simulink model "SatelliteServicing_Mission"  (R2023a)
settings: Solver=FixedStepAuto  StartTime=0.0  StopTime=endTime  FixedStep=stepSize  RelTol=1e-3  EnableMultiTasking=on
values from neighbouring files (symbols this model uses):
  nsat = 4    [loadCubesatParams.m]
undefined symbols (not defined in the file or in its folder): arm, client, cubesat, orbit, smiData, X, Y, Z
libraries: nesl_utility x53, sm_lib x32
(part 1 of 2)
settings Model: Creator=Andy  LastModifiedBy=Andy
settings SolverCC: PositivePriorityOrder=on
settings OptimizationCC: EnhancedBackFolding=on  PassReuseOutputArgsAs=Individual arguments  OptimizeBlockOrder=speed  DifferentSizesBufferReuse=on  OptimizationCustomize=off  EfficientTunableParamExpr=on
settings DebuggingCC: ParameterTunabilityLossMsg=error  UnconnectedInputMsg=warning  UnconnectedOutputMsg=warning  UnconnectedLineMsg=warning
settings ModelReferenceCC: EnableRefExpFcnMdlSchedulingChecks=on
settings SFSimCC: MATLABDynamicMemAlloc=off  SimTargetLang=C++
settings RTWCC: Description=Embedded Coder  SystemTargetFile=ert.tlc  GenCodeOnly=on  PackageGeneratedCodeAndArtifacts=on  TemplateMakefile=ert_default_tmf  GenerateReport=on  Toolchain=GNU GCC Embedded Linux  BuildConfiguration=Faster Runs  LaunchReport=on  TargetLang=C++  DLArmComputeVersion=19.05
settings CodeAppCC: ForceParamTrailComments=on  IgnoreCustomStorageClasses=off  OperatorAnnotations=on  SimulinkDataObjDesc=on  SFDataObjDesc=on  InsertBlockDesc=on
settings ERTTargetCC: TargetLangStandard=C++11 (ISO)  UtilityFuncGeneration=Shared location  GenerateSampleERTMain=on  CodeInterfacePackaging=Reusable function  SupportContinuousTime=on  SupportVariableSizeSignals=on  GenerateAllocFcn=on  RootIOFormat=Structure reference  ERTCustomFileTemplate=example_file_process.tlc
settings SimscapeCC: SimscapeLogType=all

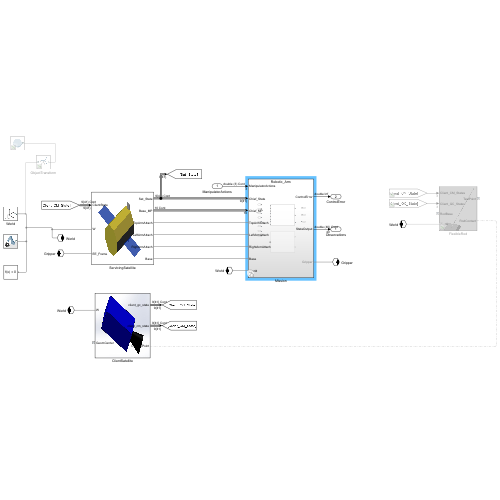
[thumbnail: Simulink's stored preview of the top-level diagram]
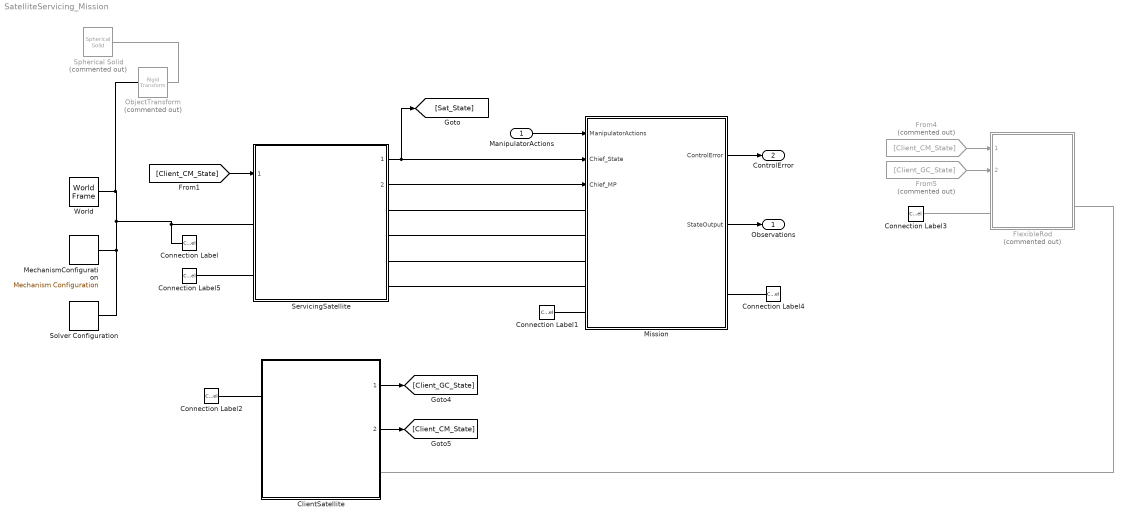
== system SatelliteServicing_Mission ==
  ManipulatorActions : Inport  PortDimensions=nAction
  ClientSatellite : Subsystem  ReferencedSubsystem=ClientSatellite
  Connection Label{,1..3} (4 alike) : ConnectionLabel  Label=World
  Connection Label4 : ConnectionLabel  Label=Gripper
  Connection Label5 : ConnectionLabel  Label=Gripper
  FlexibleRod : Subsystem  Commented=on  ReferencedSubsystem=FlexibleRodModel
  From4 : From  Commented=on  GotoTag=Client_CM_State
  From5 : From  Commented=on  GotoTag=Client_GC_State
  MechanismConfiguration : sm_lib/Utilities/Mechanism Configuration  UniformGravity=Constant  GravityVector=[0 0 -9.80665]*0  GravityVectorUnits=m/s^2  LinearizationDelta=0.001  JointModeTransitionNonlinearIterations=2
  Mission : Subsystem  Variant=on  VariantControl=Choice
  ObjectTransform : sm_lib/Frames and Transforms/Rigid Transform  Commented=on  TranslationMethod=Cartesian  TranslationStandardOffset=0  TranslationStandardOffsetUnits=m  TranslationStandardAxis=+Z  TranslationCartesianOffset=[0 -0.6 0]  TranslationCartesianOffsetUnits=m  TranslationROffset=0  TranslationROffsetUnits=m  TranslationZOffset=0  TranslationZOffsetUnits=m  TranslationThetaOffset=0  TranslationThetaOffsetUnits=deg  RotationMethod=None  RotationAngleUnits=rad  RotationStandardAxis=+Z  RotationAngle=smiData.RigidTransform(21).angle  RotationArbitraryAxis=smiData.RigidTransform(21).axis  FollAlignAxisA=+X  BaseAlignAxisA=+Y  FollAlignAxisB=+Y  BaseAlignAxisB=+Z  RotationSequenceAxes=FollowerAxes  RotationSequence=XYZ  RotationSequenceAngles=[0 0 0]  RotationSequenceAnglesUnits=rad  RotationMatrix=[1 0 0; 0 1 0; 0 0 1]  Quaternion=[1 0 0 0]
  ServicingSatellite : Subsystem  ReferencedSubsystem=ServicingSatellite
  Solver Configuration : nesl_utility/Solver Configuration  PhysicalDomain=network_engine_domain  SubClassName=solver  LeftPortType=input  RightPortType=generic  Tones=[]  Harmonics=[]  SimulateNoise=off  Profile=off  UseLocalSampling=off  EnableSwitchedLinearOptims=on  FrequencyDomain=off  UseCCode=off  RelTol=0.001  AbsTol=1e-06  MinStep=1e-09  ToWorkspace=off  RevertToSquareIcSolve=off  NumHomotopyIterations=100  PhasorMode=off  PhasorModeNumHarmonics=1  ConsistencySolver=NEWTON_FTOL  IndexReductionMethod=DerivativeReplacement  DoDC=off  ResidualTolerance=1e-09  ConsistencyTolSource=GLOBAL  ConsistencyAbsTol=0.001  ConsistencyRelTol=0.001  ConsistencyTolFactor=0.001  UseLocalSolver=off  LocalSolverChoice=NE_BACKWARD_EULER_ADVANCER  ResolveIndetEquations=on  FunctionEvalNumThread=1  LocalSolverSampleTime=0.001  DoFixedCost=off  MaxNonlinIter=3  MaxModeIter=2  ComputeImpulses=off  ImpulseIterations=2  LinearAlgebra=auto  LinearAlgebraNumThread=0  EquationFormulation=NE_TIME_EF  DelaysMemoryBudget=1024  AutomaticFiltering=on  FilteringTimeConstant=0.001  PartitionStorageMethod=AS_NEEDED  PartitionMemoryBudget=1024  PartitionMethod=ROBUST
  Spherical Solid : sm_lib/Body Elements/Spherical Solid  Commented=on  GraphicAmbientColor=[0.15 0.15 0.15 1.0]  BasedOnType=Density  CenterOfMass=[0 0 0]  CenterOfMassUnits=m  GraphicDiffuseColor=[0.5 0.5 0.5]  Density=1000  DensityUnits=kg/m^3  DoExposeReferenceFrame=on  GraphicEmissiveColor=[0.0 0.0 0.0 1.0]  ExportEntireGeometry=off  SerializedExposedGeometries=<ExposedGeometries/>  SerializedFrames=<Frames/>  MarkerShape=Sphere  MarkerSize=10  GraphicType=FromGeometry  InertiaType=CalculateFromGeometry  Mass=1  MassUnits=kg  MomentsOfInertia=[1 1 1]  MomentsOfInertiaUnits=kg*m^2  GraphicOpacity=1.0  ProductsOfInertia=[0 0 0]  ProductsOfInertiaUnits=kg*m^2  GraphicShininess=75  GraphicSpecularColor=[0.5 0.5 0.5 1.0]  SphereRadius=0.1  SphereRadiusUnits=m  GraphicVisPropType=SimpleVisualProperties
  World : sm_lib/Frames and Transforms/World Frame
  Observations : Outport
  ControlError : Outport  Port=2
  wires:
  ServicingSatellite/1 -> [Sat_State], Mission/2(Chief_State)
  ClientSatellite/1 -> [Client_GC_State]
  ClientSatellite/2 -> [Client_CM_State]
  ManipulatorActions/1 -> Mission/1(ManipulatorActions)
  Mission/1(ControlError) -> ControlError/1
  Mission/2(StateOutput) -> Observations/1
  From5/1 -> FlexibleRod/2
  From4/1 -> FlexibleRod/1
  [Client_CM_State] -> ServicingSatellite/1
  ServicingSatellite/2 -> Mission/3(Chief_MP)
  connections:
  MechanismConfiguration/RConn1 -- ServicingSatellite/LConn1 -- Connection Label/LConn1 -- ObjectTransform/LConn1 -- World/RConn1 -- Solver Configuration/RConn1
  FlexibleRod/RConn2 -- ClientSatellite/RConn1
  Connection Label2/LConn1 -- ClientSatellite/LConn1
  FlexibleRod/LConn2 -- Connection Label3/LConn1
  Mission/LConn1 -- ServicingSatellite/RConn1
  Mission/LConn4 -- ServicingSatellite/RConn4
  Mission/LConn5 -- Connection Label1/LConn1
  Connection Label4/LConn1 -- Mission/RConn1
  Connection Label5/LConn1 -- ServicingSatellite/LConn2
  ServicingSatellite/RConn2 -- Mission/LConn2
  ServicingSatellite/RConn3 -- Mission/LConn3
  Spherical Solid/RConn1 -- ObjectTransform/RConn1

== system SatelliteServicing_Mission/Mission ==
  ManipulatorActions : Inport
  Chief_State : Inport  Port=2
  Chief_MP : Inport  Port=3
  Cubesat_Inspection : Subsystem  VariantControl=VSS_CubeSatOperation
  Robotic_Arm : Subsystem  VariantControl=VSS_RoboticArmOperation
  Gripper : PMIOPort  Side=Right
  TopArmAttach : PMIOPort  Port=2  Side=Left
  LeftArmAttach : PMIOPort  Port=3  Side=Left
  RightArmAttach : PMIOPort  Port=4  Side=Left
  Base : PMIOPort  Port=5  Side=Left
  World : PMIOPort  Port=6  Side=Left
  ControlError : Outport
  StateOutput : Outport  Port=2

== system SatelliteServicing_Mission/Mission/Cubesat_Inspection ==
  Bus Selector : BusSelector  OutputSignals=Cubesat1_RelState.Rel_Position,Cubesat1_RelState.Rel_Velocity,Cubesat1_RelState.Rel_Acceleration,Cubesat2_RelState.Rel_Position,Cubesat2_RelState.Rel_Velocity,Cubesat2_RelState.Rel_Acceleration,Cubesat3_RelState.Rel_Position,Cubesat3_RelState.Rel_Velocity,Cubesat3_RelState.Rel_Acceleration,Cubesat4_RelState.Rel_Position,Cubesat4_RelState.Rel_Velocity,Cubesat4_RelState.Rel_Acceleration
  Cubesats : Subsystem
  InspectionCoverage : Subsystem
  Mux1 : Mux  Inputs=12
  To Workspace1 : ToWorkspace  VariableName=cubesatRelState  SaveFormat=Timeseries  SampleTime=-1
  World : PMIOPort  Side=Left
  StateOutput : Outport
  ControlError : Outport  Port=2
  wires:
  Cubesats/1(Cubesat_RelState) -> Bus Selector/1, To Workspace1/1, InspectionCoverage/1(relative_state)
  InspectionCoverage/1(coverageCredit) -> ControlError/1
  Mux1/1 -> StateOutput/1
  Bus Selector/1 -> Mux1/1  "<Rel_Position>"
  Bus Selector/2 -> Mux1/2  "<Rel_Velocity>"
  Bus Selector/3 -> Mux1/3  "<Rel_Acceleration>"
  Bus Selector/4 -> Mux1/4  "<Rel_Position>"
  Bus Selector/5 -> Mux1/5  "<Rel_Velocity>"
  Bus Selector/6 -> Mux1/6  "<Rel_Acceleration>"
  Bus Selector/7 -> Mux1/7  "<Rel_Position>"
  Bus Selector/8 -> Mux1/8  "<Rel_Velocity>"
  Bus Selector/9 -> Mux1/9  "<Rel_Acceleration>"
  Bus Selector/10 -> Mux1/10  "<Rel_Position>"
  Bus Selector/11 -> Mux1/11  "<Rel_Velocity>"
  Bus Selector/12 -> Mux1/12  "<Rel_Acceleration>"
  connections:
  World/RConn1 -- Cubesats/LConn1

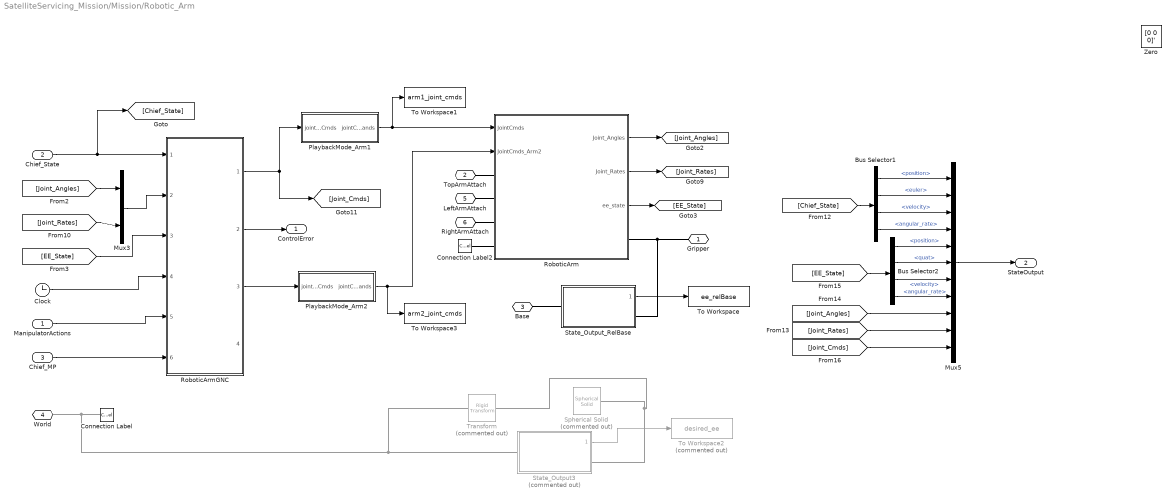
== system SatelliteServicing_Mission/Mission/Robotic_Arm ==
  ManipulatorActions : Inport  PortDimensions=nAction
  Chief_State : Inport  Port=2
  Chief_MP : Inport  Port=3
  Bus Selector1 : BusSelector  OutputSignals=translation.position,rotation.euler,translation.velocity,rotation.angular_rate
  Bus Selector2 : BusSelector  OutputSignals=translation.position,rotation.quat,translation.velocity,rotation.angular_rate
  Clock : Clock
  Connection Label : ConnectionLabel  Label=World
  Connection Label2 : ConnectionLabel  Label=World
  Mux3 : Mux  Inputs=2
  Mux5 : Mux  Inputs=11
  PlaybackMode_Arm1 : Subsystem  Variant=on  VariantControl=Choice
  PlaybackMode_Arm2 : Subsystem  Variant=on  VariantControl=Choice
  RoboticArm : Subsystem  Variant=on  VariantControl=Choice
  RoboticArmGNC : Subsystem  SystemSampleTime=0.001  ReferencedSubsystem=RoboticArmGNC
      settings: MinAlgLoopOccurrences=on
  Spherical Solid : sm_lib/Body Elements/Spherical Solid  Commented=on  GraphicAmbientColor=[0.15 0.15 0.15 1.0]  BasedOnType=Density  CenterOfMass=[0 0 0]  CenterOfMassUnits=m  GraphicDiffuseColor=[1.0 0.0 0.0]  Density=1000  DensityUnits=kg/m^3  DoExposeReferenceFrame=on  GraphicEmissiveColor=[0.0 0.0 0.0 1.0]  ExportEntireGeometry=off  SerializedExposedGeometries=<ExposedGeometries/>  SerializedFrames=<Frames/>  MarkerShape=Sphere  MarkerSize=10  GraphicType=FromGeometry  InertiaType=CalculateFromGeometry  Mass=1  MassUnits=kg  MomentsOfInertia=[1 1 1]  MomentsOfInertiaUnits=kg*m^2  GraphicOpacity=1.0  ProductsOfInertia=[0 0 0]  ProductsOfInertiaUnits=kg*m^2  GraphicShininess=75  GraphicSpecularColor=[0.5 0.5 0.5 1.0]  SphereRadius=0.01  SphereRadiusUnits=m  GraphicVisPropType=SimpleVisualProperties
  State_Output3 : Subsystem  Commented=on  ReferencedSubsystem=Collect_State_Output
  State_Output_RelBase : Subsystem  ReferencedSubsystem=Collect_State_Output_BaseFrame
  To Workspace : ToWorkspace  VariableName=ee_relBase  SaveFormat=Timeseries  SampleTime=-1
  To Workspace1 : ToWorkspace  VariableName=arm1_joint_cmds  SaveFormat=Timeseries  SampleTime=-1
  To Workspace2 : ToWorkspace  Commented=on  VariableName=desired_ee  SaveFormat=Timeseries  SampleTime=-1
  To Workspace3 : ToWorkspace  VariableName=arm2_joint_cmds  SaveFormat=Timeseries  SampleTime=-1
  Transform : sm_lib/Frames and Transforms/Rigid Transform  Commented=on  TranslationMethod=Cartesian  TranslationStandardOffset=0  TranslationStandardOffsetUnits=mm  TranslationStandardAxis=+Z  TranslationCartesianOffset=desired_ee_world_pos  TranslationCartesianOffsetUnits=m  TranslationROffset=0  TranslationROffsetUnits=m  TranslationZOffset=0  TranslationZOffsetUnits=m  TranslationThetaOffset=0  TranslationThetaOffsetUnits=deg  RotationMethod=RotationSequence  RotationAngleUnits=rad  RotationStandardAxis=+Z  RotationAngle=arm(1).smiData.RigidTransform(2).angle  RotationArbitraryAxis=desired_  FollAlignAxisA=+X  BaseAlignAxisA=+Y  FollAlignAxisB=+Y  BaseAlignAxisB=+Z  RotationSequenceAxes=FollowerAxes  RotationSequence=XYZ  RotationSequenceAngles=desired_ee_world_ori  RotationSequenceAnglesUnits=rad  RotationMatrix=[1 0 0; 0 1 0; 0 0 1]  Quaternion=[1 0 0 0]
  Zero : Constant  Value=[0 0 0]'
  Gripper : PMIOPort  Side=Right
  TopArmAttach : PMIOPort  Port=2  Side=Left
  Base : PMIOPort  Port=3  Side=Left
  World : PMIOPort  Port=4  Side=Left
  LeftArmAttach : PMIOPort  Port=5  Side=Left
  RightArmAttach : PMIOPort  Port=6  Side=Left
  ControlError : Outport
  StateOutput : Outport  Port=2
  wires:
  RoboticArm/2(Joint_Rates) -> [Joint_Rates]
  Chief_State/1 -> [Chief_State], RoboticArmGNC/1
  RoboticArm/3(ee_state) -> [EE_State]
  RoboticArm/1(Joint_Angles) -> [Joint_Angles]
  ManipulatorActions/1 -> RoboticArmGNC/5
  State_Output_RelBase/1 -> To Workspace/1
  [EE_State] -> RoboticArmGNC/3
  Clock/1 -> RoboticArmGNC/4
  RoboticArmGNC/2 -> ControlError/1
  PlaybackMode_Arm1/1(jointCommands) -> RoboticArm/1(JointCmds), To Workspace1/1
  Bus Selector1/1 -> Mux5/1  "<position>"
  [Joint_Cmds] -> Mux5/11
  [Joint_Angles] -> Mux5/9
  Bus Selector2/1 -> Mux5/5  "<position>"
  Bus Selector1/3 -> Mux5/3  "<velocity>"
  Bus Selector1/2 -> Mux5/2  "<euler>"
  Bus Selector1/4 -> Mux5/4  "<angular_rate>"
  Bus Selector2/2 -> Mux5/6  "<quat>"
  Bus Selector2/4 -> Mux5/8  "<angular_rate>"
  Mux5/1 -> StateOutput/1
  Bus Selector2/3 -> Mux5/7  "<velocity>"
  [Chief_State] -> Bus Selector1/1
  [Joint_Rates] -> Mux5/10
  [EE_State] -> Bus Selector2/1
  Chief_MP/1 -> RoboticArmGNC/6
  RoboticArmGNC/1 -> [Joint_Cmds], PlaybackMode_Arm1/1(jointTorqueCmds)
  State_Output3/1 -> To Workspace2/1
  RoboticArmGNC/3 -> PlaybackMode_Arm2/1(jointTorqueCmds)
  PlaybackMode_Arm2/1(jointCommands) -> To Workspace3/1, RoboticArm/2(JointCmds_Arm2)
  [Joint_Angles] -> Mux3/1
  [Joint_Rates] -> Mux3/2
  Mux3/1 -> RoboticArmGNC/2
  connections:
  State_Output_RelBase/RConn1 -- RoboticArm/RConn1 -- Gripper/RConn1
  Base/RConn1 -- State_Output_RelBase/LConn1
  RoboticArm/LConn1 -- TopArmAttach/RConn1
  Connection Label2/LConn1 -- RoboticArm/LConn4
  LeftArmAttach/RConn1 -- RoboticArm/LConn2
  RightArmAttach/RConn1 -- RoboticArm/LConn3
  State_Output3/LConn1 -- Connection Label/LConn1 -- World/RConn1 -- Transform/LConn1
  State_Output3/RConn1 -- Transform/RConn1 -- Spherical Solid/RConn1

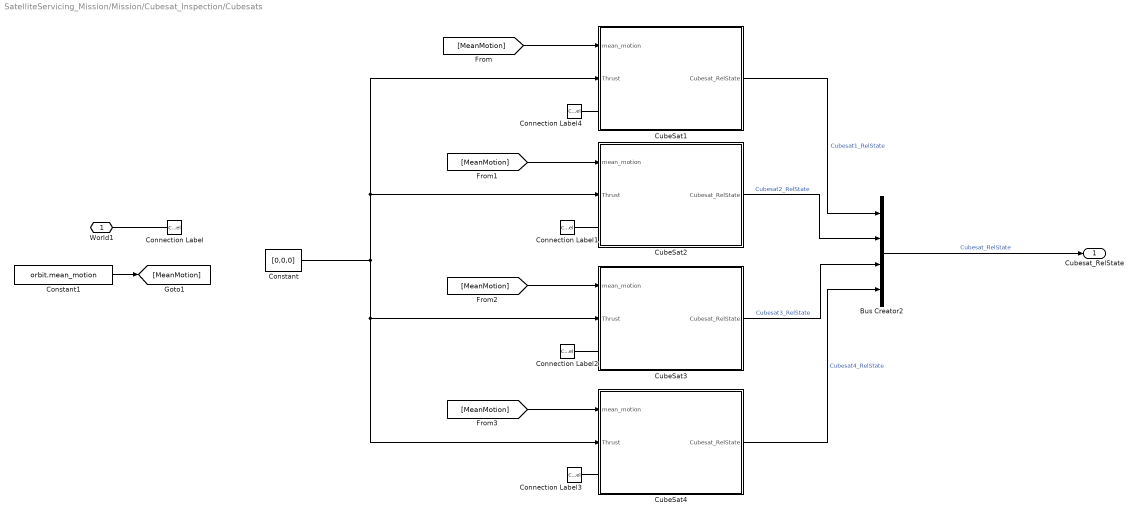
== system SatelliteServicing_Mission/Mission/Cubesat_Inspection/Cubesats ==
  Bus Creator2 : BusCreator  Inputs=4
  Connection Label{,1..4} (5 alike) : ConnectionLabel  Label=World
  Constant : Constant  Value=[0,0,0]
  Constant1 : Constant  Value=orbit.mean_motion
  CubeSat1 : Subsystem  Variant=on  VariantControl=Choice  AllowZeroVariantControls=on
  CubeSat2 : Subsystem  Variant=on  VariantControl=Choice  AllowZeroVariantControls=on
  CubeSat3 : Subsystem  Variant=on  VariantControl=Choice  AllowZeroVariantControls=on
  CubeSat4 : Subsystem  Variant=on  VariantControl=Choice  AllowZeroVariantControls=on
  World1 : PMIOPort  Side=Left
  Cubesat_RelState : Outport
  wires:
  CubeSat3/1(Cubesat_RelState) -> Bus Creator2/3  "Cubesat3_RelState"
  Constant1/1 -> [MeanMotion]
  CubeSat2/1(Cubesat_RelState) -> Bus Creator2/2  "Cubesat2_RelState"
  CubeSat4/1(Cubesat_RelState) -> Bus Creator2/4  "Cubesat4_RelState"
  [MeanMotion] -> CubeSat3/1(mean_motion)
  [MeanMotion] -> CubeSat4/1(mean_motion)
  Bus Creator2/1 -> Cubesat_RelState/1  "Cubesat_RelState"
  CubeSat1/1(Cubesat_RelState) -> Bus Creator2/1  "Cubesat1_RelState"
  Constant/1 -> CubeSat1/2(Thrust), CubeSat2/2(Thrust), CubeSat4/2(Thrust), CubeSat3/2(Thrust)
  [MeanMotion] -> CubeSat1/1(mean_motion)
  [MeanMotion] -> CubeSat2/1(mean_motion)
  connections:
  Connection Label2/LConn1 -- CubeSat3/LConn1
  World1/RConn1 -- Connection Label/LConn1
  Connection Label4/LConn1 -- CubeSat1/LConn1
  Connection Label3/LConn1 -- CubeSat4/LConn1
  Connection Label1/LConn1 -- CubeSat2/LConn1

== system SatelliteServicing_Mission/Mission/Cubesat_Inspection/InspectionCoverage ==
  relative_state : Inport
  Constant1 : Constant  Value=nsat
  Constant2 : Constant  Value=client.inspectionFOV
  Constant3 : Constant  Value=client.faceCenter
  Constant4 : Constant  Value=zeros(client.nFaces,1)  VectorParams1D=off
  Constant5 : Constant  Value=client.faceRadius
  Constant6 : Constant  Value=client.inspectionSphereRadius
  Delay : Delay  DelayLength=1  InitialConditionSource=Input port
      settings: InputPortMap=u0,p4
  Delay1 : Delay  DelayLength=1  InitialConditionSource=Input port
      settings: InputPortMap=u0,p4
  Reshape : Reshape  OutputDimensionality=Column vector (2-D)
  To Workspace7 : ToWorkspace  VariableName=coverageOut  SaveFormat=Timeseries  SampleTime=-1
  To Workspace8 : ToWorkspace  VariableName=creditOut  SaveFormat=Timeseries  SampleTime=-1
  computeCoverage : MATLAB Function  TreatAsAtomicUnit=on
  coverageCredit : Outport
  wires:
  computeCoverage/2(credit_out) -> To Workspace8/1, Delay1/1, coverageCredit/1
  Constant6/1 -> computeCoverage/6(inspectionSphereRadius)
  Constant3/1 -> computeCoverage/4(clientFaces)
  computeCoverage/1(coverage_out) -> Delay/1, To Workspace7/1
  Constant1/1 -> computeCoverage/1(nsat)
  Constant4/1 -> Delay1/2, Delay/2
  Constant5/1 -> computeCoverage/5(faceRadius)
  Delay/1 -> computeCoverage/7(coverage_in)
  relative_state/1 -> Reshape/1
  Constant2/1 -> computeCoverage/3(fov)
  Delay1/1 -> computeCoverage/8(credit_in)
  Reshape/1 -> computeCoverage/2(relative_state)

== system SatelliteServicing_Mission/Mission/Robotic_Arm/PlaybackMode_Arm1 ==
  jointTorqueCmds : Inport  PortDimensions=nLink
  Computed_JointTorques : Subsystem  VariantControl=(default)
  Playback_JointAngles : Subsystem  VariantControl=ARM1_CONTROL_TYPE == 4
  jointCommands : Outport

== system SatelliteServicing_Mission/Mission/Robotic_Arm/PlaybackMode_Arm2 ==
  jointTorqueCmds : Inport  PortDimensions=nLink
  Computed_JointTorques : Subsystem  VariantControl=(default)
  Playback_JointAngles : Subsystem  VariantControl=ARM2_CONTROL_TYPE == 4
  jointCommands : Outport

== system SatelliteServicing_Mission/Mission/Robotic_Arm/RoboticArm ==
  JointCmds : Inport
  JointCmds_Arm2 : Inport  Port=2
  RoboticArmDualArms3DOF : Subsystem  VariantControl=VSS_RoboticArmDualArm3DOF
  RoboticArmDualArms7DOF : Subsystem  VariantControl=VSS_RoboticArmDualArm7DOF
  RoboticArmGeneral6DOF : Subsystem  VariantControl=VSS_RoboticArmGeneral6DOF  ReferencedSubsystem=RoboticArmGeneral6DOF
  RoboticArmGeneral7DOF : Subsystem  VariantControl=VSS_RoboticArmGeneral7DOF  ReferencedSubsystem=RoboticArmGeneral7DOF_1  armAttach_Data=0  joint1_Data=0  joint2_Data=0  joint3_Data=0  joint4_Data=0  joint5_Data=0  joint6_Data=0  joint7_Data=0  ee_State_Data=0
  RoboticArmPlanar2Link : Subsystem  VariantControl=VSS_RoboticArmPlanar2Link  ReferencedSubsystem=RoboticArmPlanar2Link
  RoboticArmPlanar3Link : Subsystem  VariantControl=VSS_RoboticArmPlanar3Link  ReferencedSubsystem=RoboticArmPlanar3Link_1
  RoboticArmViperX300 : Subsystem  VariantControl=VSS_RoboticArmViperX300  ReferencedSubsystem=RoboticArmViperX300
  Gripper : PMIOPort  Side=Right
  ArmAttach : PMIOPort  Port=2  Side=Left
  LeftArmAttach : PMIOPort  Port=3  Side=Left
  RightArmAttach : PMIOPort  Port=4  Side=Left
  World : PMIOPort  Port=5  Side=Left
  Joint_Angles : Outport
  Joint_Rates : Outport  Port=2
  ee_state : Outport  Port=3

== system SatelliteServicing_Mission/Mission/Cubesat_Inspection/Cubesats/CubeSat1 ==
  mean_motion : Inport
  Thrust : Inport  Port=2
  CubeSat1_Propagation : Subsystem  VariantControl=nsat>0
  Zero : Subsystem  VariantControl=(default)
  World : PMIOPort  Side=Left
  Cubesat_RelState : Outport

== system SatelliteServicing_Mission/Mission/Cubesat_Inspection/Cubesats/CubeSat2 ==
  mean_motion : Inport
  Thrust : Inport  Port=2
  CubeSat2_Propagation : Subsystem  VariantControl=nsat>1
  Zero : Subsystem  VariantControl=(default)
  World : PMIOPort  Side=Left
  Cubesat_RelState : Outport

== system SatelliteServicing_Mission/Mission/Cubesat_Inspection/Cubesats/CubeSat3 ==
  mean_motion : Inport
  Thrust : Inport  Port=2
  CubeSat3_Propagation : Subsystem  VariantControl=nsat>2
  Zero : Subsystem  VariantControl=(default)
  World : PMIOPort  Side=Left
  Cubesat_RelState : Outport

== system SatelliteServicing_Mission/Mission/Cubesat_Inspection/Cubesats/CubeSat4 ==
  mean_motion : Inport
  Thrust : Inport  Port=2
  CubeSat4_Propagation : Subsystem  VariantControl=nsat>3
  Zero : Subsystem  VariantControl=(default)
  World : PMIOPort  Side=Left
  Cubesat_RelState : Outport

== system SatelliteServicing_Mission/Mission/Robotic_Arm/PlaybackMode_Arm1/Computed_JointTorques ==
  jointTorqueCmds : Inport  PortDimensions=nLink
  jointCommands : Outport
  wires:
  jointTorqueCmds/1 -> jointCommands/1

== system SatelliteServicing_Mission/Mission/Robotic_Arm/PlaybackMode_Arm1/Playback_JointAngles ==
  From Workspace : FromWorkspace  VariableName=prescribed_jointAngles  OutputAfterFinalValue=Holding final value
  jointCommands : Outport
  wires:
  From Workspace/1 -> jointCommands/1

== system SatelliteServicing_Mission/Mission/Robotic_Arm/PlaybackMode_Arm2/Computed_JointTorques ==
  jointTorqueCmds : Inport  PortDimensions=nLink
  jointCommands : Outport
  wires:
  jointTorqueCmds/1 -> jointCommands/1

== system SatelliteServicing_Mission/Mission/Robotic_Arm/PlaybackMode_Arm2/Playback_JointAngles ==
  From Workspace : FromWorkspace  VariableName=prescribed_jointAngles  OutputAfterFinalValue=Holding final value
  jointCommands : Outport
  wires:
  From Workspace/1 -> jointCommands/1

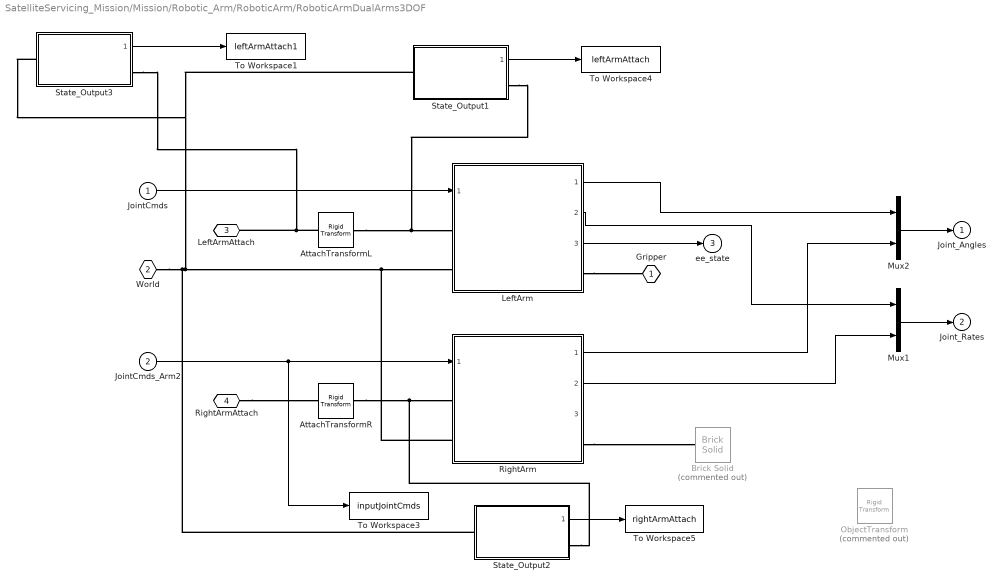
== system SatelliteServicing_Mission/Mission/Robotic_Arm/RoboticArm/RoboticArmDualArms3DOF ==
  JointCmds : Inport
  JointCmds_Arm2 : Inport  Port=2
  AttachTransformL : sm_lib/Frames and Transforms/Rigid Transform  TranslationMethod=Cartesian  TranslationStandardOffset=0  TranslationStandardOffsetUnits=m  TranslationStandardAxis=+Z  TranslationCartesianOffset=arm(1).armAttachOffset(1).translation  TranslationCartesianOffsetUnits=m  TranslationROffset=0  TranslationROffsetUnits=m  TranslationZOffset=0  TranslationZOffsetUnits=m  TranslationThetaOffset=0  TranslationThetaOffsetUnits=deg  RotationMethod=RotationSequence  RotationAngleUnits=rad  RotationStandardAxis=+Z  RotationAngle=smiData.RigidTransform(21).angle  RotationArbitraryAxis=smiData.RigidTransform(21).axis  FollAlignAxisA=+X  BaseAlignAxisA=+Y  FollAlignAxisB=+Y  BaseAlignAxisB=+Z  RotationSequenceAxes=FollowerAxes  RotationSequence=XYZ  RotationSequenceAngles=arm(1).armAttachOffset(1).orientation  RotationSequenceAnglesUnits=rad  RotationMatrix=[1 0 0; 0 1 0; 0 0 1]  Quaternion=[1 0 0 0]
  AttachTransformR : sm_lib/Frames and Transforms/Rigid Transform  TranslationMethod=Cartesian  TranslationStandardOffset=0  TranslationStandardOffsetUnits=m  TranslationStandardAxis=+Z  TranslationCartesianOffset=arm(2).armAttachOffset(1).translation  TranslationCartesianOffsetUnits=m  TranslationROffset=0  TranslationROffsetUnits=m  TranslationZOffset=0  TranslationZOffsetUnits=m  TranslationThetaOffset=0  TranslationThetaOffsetUnits=deg  RotationMethod=RotationSequence  RotationAngleUnits=rad  RotationStandardAxis=+Z  RotationAngle=smiData.RigidTransform(21).angle  RotationArbitraryAxis=smiData.RigidTransform(21).axis  FollAlignAxisA=+X  BaseAlignAxisA=+Y  FollAlignAxisB=+Y  BaseAlignAxisB=+Z  RotationSequenceAxes=FollowerAxes  RotationSequence=XYZ  RotationSequenceAngles=arm(2).armAttachOffset(1).orientation  RotationSequenceAnglesUnits=rad  RotationMatrix=[1 0 0; 0 1 0; 0 0 1]  Quaternion=[1 0 0 0]
  Brick Solid : sm_lib/Body Elements/Brick Solid  Commented=on  GraphicAmbientColor=[0.15 0.15 0.15 1.0]  BasedOnType=Mass  BrickDimensions=[0.1 0.1 0.2]  BrickDimensionsUnits=m  CenterOfMass=[0 0 0]  CenterOfMassUnits=m  GraphicDiffuseColor=[0.2 0.8 0.0]  Density=1000  DensityUnits=kg/m^3  DoExposeReferenceFrame=on  GraphicEmissiveColor=[0.0 0.0 0.0 1.0]  ExportEntireGeometry=off  SerializedFrames=<Frames/>  MarkerShape=Sphere  MarkerSize=10  GraphicType=FromGeometry  InertiaType=CalculateFromGeometry  Mass=3  MassUnits=kg  MomentsOfInertia=[1 1 1]  MomentsOfInertiaUnits=kg*m^2  GraphicOpacity=1.0  ProductsOfInertia=[0 0 0]  ProductsOfInertiaUnits=kg*m^2  GraphicShininess=75  GraphicSpecularColor=[0.5 0.5 0.5 1.0]  GraphicVisPropType=SimpleVisualProperties
  LeftArm : Subsystem  ReferencedSubsystem=RoboticArmPlanar3Link_1
  Mux1 : Mux  Inputs=2
  Mux2 : Mux  Inputs=2
  ObjectTransform : sm_lib/Frames and Transforms/Rigid Transform  Commented=on  TranslationMethod=Cartesian  TranslationStandardOffset=0  TranslationStandardOffsetUnits=m  TranslationStandardAxis=+Z  TranslationCartesianOffset=[0 -0.6 0]  TranslationCartesianOffsetUnits=m  TranslationROffset=0  TranslationROffsetUnits=m  TranslationZOffset=0  TranslationZOffsetUnits=m  TranslationThetaOffset=0  TranslationThetaOffsetUnits=deg  RotationMethod=None  RotationAngleUnits=rad  RotationStandardAxis=+Z  RotationAngle=smiData.RigidTransform(21).angle  RotationArbitraryAxis=smiData.RigidTransform(21).axis  FollAlignAxisA=+X  BaseAlignAxisA=+Y  FollAlignAxisB=+Y  BaseAlignAxisB=+Z  RotationSequenceAxes=FollowerAxes  RotationSequence=XYZ  RotationSequenceAngles=[0 0 0]  RotationSequenceAnglesUnits=rad  RotationMatrix=[1 0 0; 0 1 0; 0 0 1]  Quaternion=[1 0 0 0]
  RightArm : Subsystem  ReferencedSubsystem=RoboticArmPlanar3Link_2
  State_Output1 : Subsystem  ReferencedSubsystem=Collect_State_Output
  State_Output2 : Subsystem  ReferencedSubsystem=Collect_State_Output
  State_Output3 : Subsystem  ReferencedSubsystem=Collect_State_Output
  To Workspace1 : ToWorkspace  VariableName=leftArmAttach1  SaveFormat=Timeseries  SampleTime=-1
  To Workspace3 : ToWorkspace  VariableName=inputJointCmds  SaveFormat=Timeseries  SampleTime=-1
  To Workspace4 : ToWorkspace  VariableName=leftArmAttach  SaveFormat=Timeseries  SampleTime=-1
  To Workspace5 : ToWorkspace  VariableName=rightArmAttach  SaveFormat=Timeseries  SampleTime=-1
  Gripper : PMIOPort  Side=Right
  World : PMIOPort  Port=2  Side=Left
  LeftArmAttach : PMIOPort  Port=3  Side=Left
  RightArmAttach : PMIOPort  Port=4  Side=Left
  Joint_Angles : Outport
  Joint_Rates : Outport  Port=2
  ee_state : Outport  Port=3
  wires:
  Mux2/1 -> Joint_Angles/1
  Mux1/1 -> Joint_Rates/1
  JointCmds/1 -> LeftArm/1
  JointCmds_Arm2/1 -> To Workspace3/1, RightArm/1
  LeftArm/1 -> Mux2/1
  LeftArm/2 -> Mux1/1
  LeftArm/3 -> ee_state/1
  RightArm/1 -> Mux2/2
  RightArm/2 -> Mux1/2
  State_Output1/1 -> To Workspace4/1
  State_Output2/1 -> To Workspace5/1
  State_Output3/1 -> To Workspace1/1
  connections:
  RightArmAttach/RConn1 -- AttachTransformR/LConn1
  AttachTransformL/LConn1 -- State_Output3/RConn1 -- LeftArmAttach/RConn1
  World/RConn1 -- State_Output2/LConn1 -- State_Output3/LConn1 -- State_Output1/LConn1 -- RightArm/LConn2 -- LeftArm/LConn2
  LeftArm/RConn1 -- Gripper/RConn1
  AttachTransformR/RConn1 -- State_Output2/RConn1 -- RightArm/LConn1
  AttachTransformL/RConn1 -- State_Output1/RConn1 -- LeftArm/LConn1
  RightArm/RConn1 -- Brick Solid/RConn1

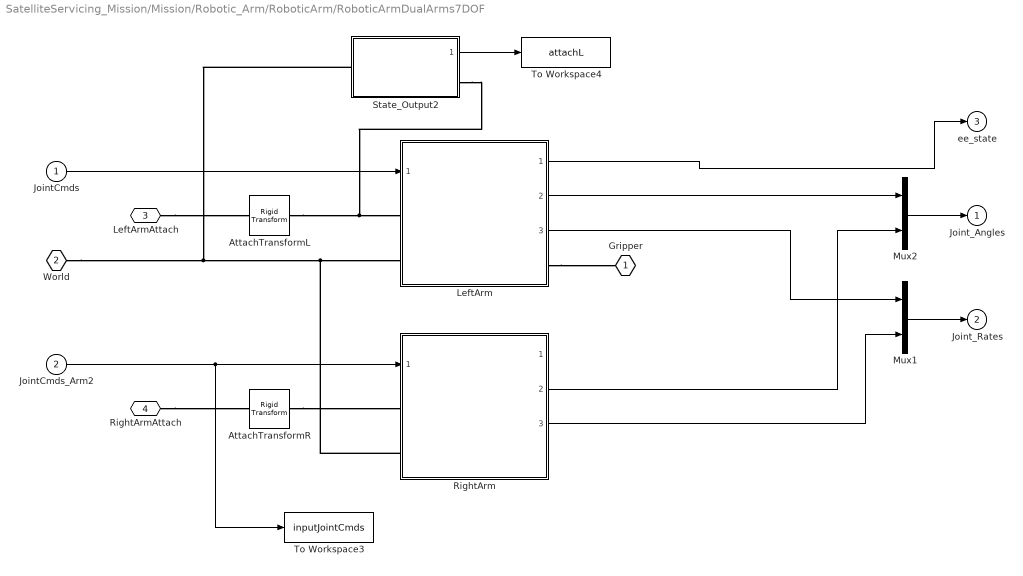
== system SatelliteServicing_Mission/Mission/Robotic_Arm/RoboticArm/RoboticArmDualArms7DOF ==
  JointCmds : Inport
  JointCmds_Arm2 : Inport  Port=2
  AttachTransformL : sm_lib/Frames and Transforms/Rigid Transform  TranslationMethod=Cartesian  TranslationStandardOffset=0  TranslationStandardOffsetUnits=m  TranslationStandardAxis=+Z  TranslationCartesianOffset=arm(1).armAttachOffset(1).translation  TranslationCartesianOffsetUnits=m  TranslationROffset=0  TranslationROffsetUnits=m  TranslationZOffset=0  TranslationZOffsetUnits=m  TranslationThetaOffset=0  TranslationThetaOffsetUnits=deg  RotationMethod=RotationSequence  RotationAngleUnits=rad  RotationStandardAxis=+Z  RotationAngle=smiData.RigidTransform(21).angle  RotationArbitraryAxis=smiData.RigidTransform(21).axis  FollAlignAxisA=+X  BaseAlignAxisA=+Y  FollAlignAxisB=+Y  BaseAlignAxisB=+Z  RotationSequenceAxes=BaseAxes  RotationSequence=ZYX  RotationSequenceAngles=arm(1).armAttachOffset(1).orientation  RotationSequenceAnglesUnits=rad  RotationMatrix=[1 0 0; 0 1 0; 0 0 1]  Quaternion=[1 0 0 0]
  AttachTransformR : sm_lib/Frames and Transforms/Rigid Transform  TranslationMethod=Cartesian  TranslationStandardOffset=0  TranslationStandardOffsetUnits=m  TranslationStandardAxis=+Z  TranslationCartesianOffset=arm(2).armAttachOffset(1).translation  TranslationCartesianOffsetUnits=m  TranslationROffset=0  TranslationROffsetUnits=m  TranslationZOffset=0  TranslationZOffsetUnits=m  TranslationThetaOffset=0  TranslationThetaOffsetUnits=deg  RotationMethod=RotationSequence  RotationAngleUnits=rad  RotationStandardAxis=+Z  RotationAngle=smiData.RigidTransform(21).angle  RotationArbitraryAxis=smiData.RigidTransform(21).axis  FollAlignAxisA=+X  BaseAlignAxisA=+Y  FollAlignAxisB=+Y  BaseAlignAxisB=+Z  RotationSequenceAxes=BaseAxes  RotationSequence=ZYX  RotationSequenceAngles=arm(2).armAttachOffset(1).orientation  RotationSequenceAnglesUnits=rad  RotationMatrix=[1 0 0; 0 1 0; 0 0 1]  Quaternion=[1 0 0 0]
  LeftArm : Subsystem  ReferencedSubsystem=RoboticArmGeneral7DOF_1  armAttach_Data='armAttach_Data1'  joint1_Data='joint1_Data1'  joint2_Data='joint2_Data1'  joint3_Data='joint3_Data1'  joint4_Data='joint4_Data1'  joint5_Data='joint5_Data1'  joint6_Data='joint6_Data1'  joint7_Data='joint7_Data1'  ee_State_Data='ee_State_Data1'
  Mux1 : Mux  Inputs=2
  Mux2 : Mux  Inputs=2
  RightArm : Subsystem  ReferencedSubsystem=RoboticArmGeneral7DOF_2  armAttach_Data='armAttach_Data2'  joint1_Data='joint1_Data2'  joint2_Data='joint2_Data2'  joint3_Data='joint3_Data2'  joint4_Data='joint4_Data2'  joint5_Data='joint5_Data2'  joint6_Data='joint6_Data2'  joint7_Data='joint7_Data2'  ee_State_Data='ee_State_Data2'
  State_Output2 : Subsystem  ReferencedSubsystem=Collect_State_Output
  To Workspace3 : ToWorkspace  VariableName=inputJointCmds  SaveFormat=Timeseries  SampleTime=-1
  To Workspace4 : ToWorkspace  VariableName=attachL  SaveFormat=Timeseries  SampleTime=-1
  Gripper : PMIOPort  Side=Right
  World : PMIOPort  Port=2  Side=Left
  LeftArmAttach : PMIOPort  Port=3  Side=Left
  RightArmAttach : PMIOPort  Port=4  Side=Left
  Joint_Angles : Outport
  Joint_Rates : Outport  Port=2
  ee_state : Outport  Port=3
  wires:
  LeftArm/2 -> Mux2/1
  RightArm/2 -> Mux2/2
  RightArm/3 -> Mux1/2
  Mux2/1 -> Joint_Angles/1
  LeftArm/3 -> Mux1/1
  Mux1/1 -> Joint_Rates/1
  LeftArm/1 -> ee_state/1
  JointCmds/1 -> LeftArm/1
  JointCmds_Arm2/1 -> To Workspace3/1, RightArm/1
  State_Output2/1 -> To Workspace4/1
  connections:
  RightArmAttach/RConn1 -- AttachTransformR/LConn1
  LeftArmAttach/RConn1 -- AttachTransformL/LConn1
  World/RConn1 -- State_Output2/LConn1 -- RightArm/LConn2 -- LeftArm/LConn2
  LeftArm/RConn1 -- Gripper/RConn1
  AttachTransformR/RConn1 -- RightArm/LConn1
  AttachTransformL/RConn1 -- State_Output2/RConn1 -- LeftArm/LConn1

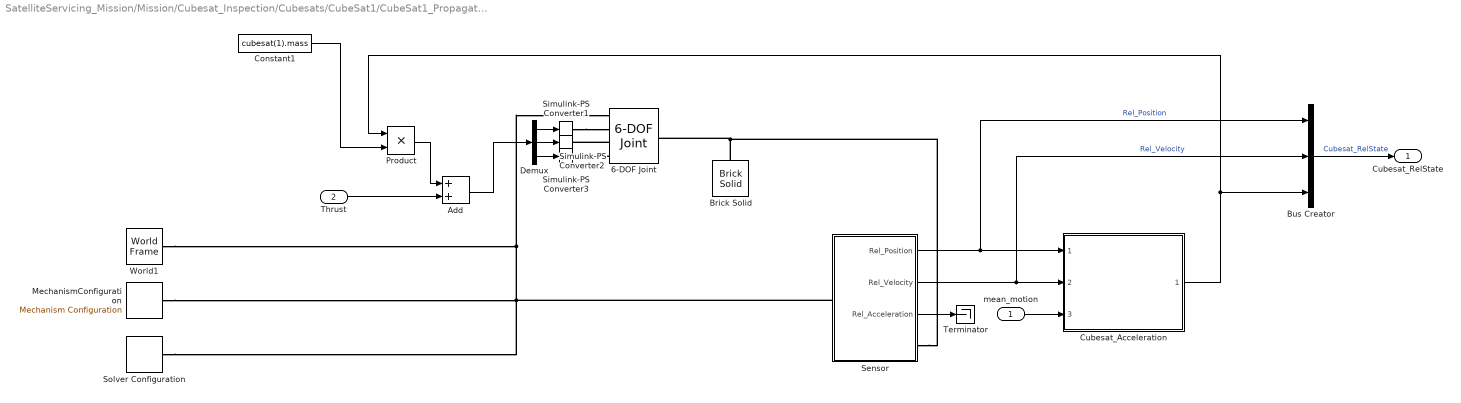
== system SatelliteServicing_Mission/Mission/Cubesat_Inspection/Cubesats/CubeSat1/CubeSat1_Propagation ==
  mean_motion : Inport
  Thrust : Inport  Port=2
  6-DOF Joint : sm_lib/Joints/6-DOF Joint  JointMode=Normal  SenseConstraintForce=off  SenseConstraintForceX=off  SenseConstraintForceY=off  SenseConstraintForceZ=off  SenseConstraintTorque=off  SenseConstraintTorqueX=off  SenseConstraintTorqueY=off  SenseConstraintTorqueZ=off  SenseTotalForce=off  SenseTotalForceX=off  SenseTotalForceY=off  SenseTotalForceZ=off  SenseTotalTorque=off  SenseTotalTorqueX=off  SenseTotalTorqueY=off  SenseTotalTorqueZ=off  CompositeWrenchDir=FollowerOnBase  CompositeWrenchFrame=BaseFrame  PxEquilibriumPosition=0  PxEquilibriumPositionUnits=m  PxSpringStiffness=0  PxSpringStiffnessUnits=N/m  PxDampingCoefficient=0  PxDampingCoefficientUnits=N/(m/s)  PxTorqueActuationMode=InputTorque  PxMotionActuationMode=ComputedMotion  PxSensePosition=off  PxSenseVelocity=off  PxSenseAcceleration=off  PxSenseTorqueForce=off  PxSenseLowerLimitTorqueForce=off  PxSenseUpperLimitTorqueForce=off  PxLowerLimitSpecify=off  PxLowerLimitBound=-1  PxLowerLimitBoundUnits=m  PxLowerLimitStiffness=1e6  PxLowerLimitStiffnessUnits=N/m  PxLowerLimitDamping=1e3  PxLowerLimitDampingUnits=N/(m/s)  PxLowerLimitTransitionRegionWidth=1e-4  PxLowerLimitTransitionRegionWidthUnits=m  PxUpperLimitSpecify=off  PxUpperLimitBound=1  PxUpperLimitBoundUnits=m  PxUpperLimitStiffness=1e6  PxUpperLimitStiffnessUnits=N/m  PxUpperLimitDamping=1e3  PxUpperLimitDampingUnits=N/(m/s)  PxUpperLimitTransitionRegionWidth=1e-4  PxUpperLimitTransitionRegionWidthUnits=m  PxPositionTargetSpecify=on  PxPositionTargetPriority=High  PxPositionTargetValue=cubesat(1).IC.rel_position(1)  PxPositionTargetValueUnits=m  PxVelocityTargetSpecify=on  PxVelocityTargetPriority=High  PxVelocityTargetValue=cubesat(1).IC.rel_velocity(1)  PxVelocityTargetValueUnits=m/s  PyEquilibriumPosition=0  PyEquilibriumPositionUnits=m  PySpringStiffness=0  PySpringStiffnessUnits=N/m  PyDampingCoefficient=0  PyDampingCoefficientUnits=N/(m/s)  PyTorqueActuationMode=InputTorque  PyMotionActuationMode=ComputedMotion  PySensePosition=off  PySenseVelocity=off  PySenseAcceleration=off  PySenseTorqueForce=off  PySenseLowerLimitTorqueForce=off  PySenseUpperLimitTorqueForce=off  PyLowerLimitSpecify=off  PyLowerLimitBound=-1  PyLowerLimitBoundUnits=m  PyLowerLimitStiffness=1e6  PyLowerLimitStiffnessUnits=N/m  PyLowerLimitDamping=1e3  PyLowerLimitDampingUnits=N/(m/s)  PyLowerLimitTransitionRegionWidth=1e-4  PyLowerLimitTransitionRegionWidthUnits=m  PyUpperLimitSpecify=off  PyUpperLimitBound=1  PyUpperLimitBoundUnits=m  PyUpperLimitStiffness=1e6  PyUpperLimitStiffnessUnits=N/m  PyUpperLimitDamping=1e3  PyUpperLimitDampingUnits=N/(m/s)  PyUpperLimitTransitionRegionWidth=1e-4  PyUpperLimitTransitionRegionWidthUnits=m  PyPositionTargetSpecify=on  PyPositionTargetPriority=High  PyPositionTargetValue=cubesat(1).IC.rel_position(2)  PyPositionTargetValueUnits=m  PyVelocityTargetSpecify=on  PyVelocityTargetPriority=High  PyVelocityTargetValue=cubesat(1).IC.rel_velocity(2)  PyVelocityTargetValueUnits=m/s  PzEquilibriumPosition=0  PzEquilibriumPositionUnits=m  PzSpringStiffness=0  PzSpringStiffnessUnits=N/m  PzDampingCoefficient=0  PzDampingCoefficientUnits=N/(m/s)  PzTorqueActuationMode=InputTorque  PzMotionActuationMode=ComputedMotion  PzSensePosition=off  PzSenseVelocity=off  PzSenseAcceleration=off  PzSenseTorqueForce=off  PzSenseLowerLimitTorqueForce=off  PzSenseUpperLimitTorqueForce=off  PzLowerLimitSpecify=off  PzLowerLimitBound=-1  PzLowerLimitBoundUnits=m  PzLowerLimitStiffness=1e6  PzLowerLimitStiffnessUnits=N/m  PzLowerLimitDamping=1e3  PzLowerLimitDampingUnits=N/(m/s)  PzLowerLimitTransitionRegionWidth=1e-4  PzLowerLimitTransitionRegionWidthUnits=m  PzUpperLimitSpecify=off  PzUpperLimitBound=1  PzUpperLimitBoundUnits=m  PzUpperLimitStiffness=1e6  PzUpperLimitStiffnessUnits=N/m  PzUpperLimitDamping=1e3  PzUpperLimitDampingUnits=N/(m/s)  PzUpperLimitTransitionRegionWidth=1e-4  PzUpperLimitTransitionRegionWidthUnits=m  PzPositionTargetSpecify=on  PzPositionTargetPriority=High  PzPositionTargetValue=cubesat(1).IC.rel_position(3)  PzPositionTargetValueUnits=m  PzVelocityTargetSpecify=on  PzVelocityTargetPriority=High  PzVelocityTargetValue=cubesat(1).IC.rel_velocity(3)  PzVelocityTargetValueUnits=m/s  SphEqPosRotationMethod=None  SphEqPosRotationAngleUnits=deg  SphEqPosRotationStandardAxis=+Z  SphEqPosRotationAngle=0.0  SphEqPosRotationArbitraryAxis=[0 0 1]  SphEqPosFollAlignAxisA=+X  SphEqPosBaseAlignAxisA=+Y  SphEqPosFollAlignAxisB=+Y  SphEqPosBaseAlignAxisB=+Z  SphEqPosRotationSequenceAxes=FollowerAxes  SphEqPosRotationSequence=XYX  SphEqPosRotationSequenceAngles=[0 0 0]  SphEqPosRotationSequenceAnglesUnits=deg  SphEqPosRotationMatrix=[1 0 0; 0 1 0; 0 0 1]  SphEqPosQuaternion=[1 0 0 0]  SphSpringStiffness=0  SphSpringStiffnessUnits=N*m/deg  SphDampingCoefficient=0  SphDampingCoefficientUnits=N*m/(deg/s)  SphActuateTorqueX=off  SphActuateTorqueY=off  SphActuateTorqueZ=off  SphActuateTorque=off  SphTorqueActuationMode=NoTorque  SphMotionActuationMode=ComputedMotion  SphActuationFrame=BaseFrame  SphSensePosition=off  SphSenseVelocityX=off  SphSenseVelocityY=off  SphSenseVelocityZ=off  SphSenseVelocity=off  SphSenseAccelerationX=off  SphSenseAccelerationY=off  SphSenseAccelerationZ=off  SphSenseAcceleration=off  SphSenseTorqueX=off  SphSenseTorqueY=off  SphSenseTorqueZ=off  SphSenseTorqueForce=off  SphSenseLowerLimitTorqueMag=off  SphSenseUpperLimitTorqueMag=off  SphSensingFrame=BaseFrame  SphLowerLimitSpecify=off  SphLowerLimitBound=15  SphLowerLimitBoundUnits=deg  SphLowerLimitStiffness=1e4  SphLowerLimitStiffnessUnits=N*m/deg  SphLowerLimitDamping=10  SphLowerLimitDampingUnits=N*m/(deg/s)  SphLowerLimitTransitionRegionWidth=0.1  SphLowerLimitTransitionRegionWidthUnits=deg  SphUpperLimitSpecify=off  SphUpperLimitBound=45  SphUpperLimitBoundUnits=deg  SphUpperLimitStiffness=1e4  SphUpperLimitStiffnessUnits=N*m/deg  SphUpperLimitDamping=10  SphUpperLimitDampingUnits=N*m/(deg/s)  SphUpperLimitTransitionRegionWidth=0.1  SphUpperLimitTransitionRegionWidthUnits=deg  SphPositionTargetRotationMethod=None  SphPositionTargetRotationAngleUnits=deg  SphPositionTargetRotationStandardAxis=+Z  SphPositionTargetRotationAngle=0.0  SphPositionTargetRotationArbitraryAxis=[0 0 1]  SphPositionTargetFollAlignAxisA=+X  SphPositionTargetBaseAlignAxisA=+Y  SphPositionTargetFollAlignAxisB=+Y  SphPositionTargetBaseAlignAxisB=+Z  SphPositionTargetRotationSequenceAxes=FollowerAxes  SphPositionTargetRotationSequence=XYX  SphPositionTargetRotationSequenceAngles=[0 0 0]  SphPositionTargetRotationSequenceAnglesUnits=deg  SphPositionTargetRotationMatrix=[1 0 0; 0 1 0; 0 0 1]  SphPositionTargetQuaternion=[1 0 0 0]  SphPositionTargetSpecify=off  SphPositionTargetPriority=High  SphVelocityTargetValue=0  SphVelocityTargetValueUnits=rad/s  SphVelocityTargetSpecify=off  SphVelocityTargetPriority=High  SphVelocityTargetInFollowerFrame=on
  Add : Sum
  Brick Solid : sm_lib/Body Elements/Brick Solid  GraphicAmbientColor=[0.15 0.15 0.15 1.0]  BasedOnType=Density  BrickDimensions=cubesat(1).dim  BrickDimensionsUnits=m  CenterOfMass=[0 0 0]  CenterOfMassUnits=m  GraphicDiffuseColor=[0.5 0.5 0.5]  Density=1000  DensityUnits=kg/m^3  DoExposeReferenceFrame=on  GraphicEmissiveColor=[0.0 0.0 0.0 1.0]  ExportEntireGeometry=off  SerializedFrames=<Frames/>  MarkerShape=Sphere  MarkerSize=10  GraphicType=FromGeometry  InertiaType=CalculateFromGeometry  Mass=1  MassUnits=kg  MomentsOfInertia=[1 1 1]  MomentsOfInertiaUnits=kg*m^2  GraphicOpacity=1.0  ProductsOfInertia=[0 0 0]  ProductsOfInertiaUnits=kg*m^2  GraphicShininess=75  GraphicSpecularColor=[0.5 0.5 0.5 1.0]  GraphicVisPropType=SimpleVisualProperties
  Bus Creator : BusCreator  Inputs=3
  Constant1 : Constant  Value=cubesat(1).mass
  Cubesat_Acceleration : Subsystem  ReferencedSubsystem=Cubesat_Acceleration
  Demux : Demux  Outputs=3
  MechanismConfiguration : sm_lib/Utilities/Mechanism Configuration  UniformGravity=Constant  GravityVector=[0 0 -9.80665]*0  GravityVectorUnits=m/s^2  LinearizationDelta=0.001  JointModeTransitionNonlinearIterations=2
  Product : Product
  Sensor : Subsystem
  Simulink-PS Converter1 : nesl_utility/Simulink-PS Converter  PhysicalDomain=network_engine_domain  SubClassName=ps_input  LeftPortType=input  RightPortType=output  PseudoPeriodic=off  Frequencies=[]  NoiseDistribution=none  NoiseParameters=[]  Unit=1  AffineConversion=off  FilteringAndDerivatives=provide  SimscapeFilterOrder=1  InputFilterTimeConstant=0.001  UdotUserProvided=0
  Simulink-PS Converter2 : nesl_utility/Simulink-PS Converter  PhysicalDomain=network_engine_domain  SubClassName=ps_input  LeftPortType=input  RightPortType=output  PseudoPeriodic=off  Frequencies=[]  NoiseDistribution=none  NoiseParameters=[]  Unit=1  AffineConversion=off  FilteringAndDerivatives=provide  SimscapeFilterOrder=1  InputFilterTimeConstant=0.001  UdotUserProvided=0
  Simulink-PS Converter3 : nesl_utility/Simulink-PS Converter  PhysicalDomain=network_engine_domain  SubClassName=ps_input  LeftPortType=input  RightPortType=output  PseudoPeriodic=off  Frequencies=[]  NoiseDistribution=none  NoiseParameters=[]  Unit=1  AffineConversion=off  FilteringAndDerivatives=provide  SimscapeFilterOrder=1  InputFilterTimeConstant=0.001  UdotUserProvided=0
  Solver Configuration : nesl_utility/Solver Configuration  PhysicalDomain=network_engine_domain  SubClassName=solver  LeftPortType=input  RightPortType=generic  Tones=[]  Harmonics=[]  SimulateNoise=off  Profile=off  UseLocalSampling=off  EnableSwitchedLinearOptims=on  FrequencyDomain=off  UseCCode=off  RelTol=0.001  AbsTol=1e-06  MinStep=1e-09  ToWorkspace=off  RevertToSquareIcSolve=off  NumHomotopyIterations=100  PhasorMode=off  PhasorModeNumHarmonics=1  ConsistencySolver=NEWTON_FTOL  IndexReductionMethod=DerivativeReplacement  DoDC=off  ResidualTolerance=1e-09  ConsistencyTolSource=GLOBAL  ConsistencyAbsTol=0.001  ConsistencyRelTol=0.001  ConsistencyTolFactor=0.001  UseLocalSolver=off  LocalSolverChoice=NE_BACKWARD_EULER_ADVANCER  ResolveIndetEquations=on  FunctionEvalNumThread=1  LocalSolverSampleTime=0.001  DoFixedCost=off  MaxNonlinIter=3  MaxModeIter=2  ComputeImpulses=off  ImpulseIterations=2  LinearAlgebra=auto  LinearAlgebraNumThread=0  EquationFormulation=NE_TIME_EF  DelaysMemoryBudget=1024  AutomaticFiltering=on  FilteringTimeConstant=0.001  PartitionStorageMethod=AS_NEEDED  PartitionMemoryBudget=1024  PartitionMethod=ROBUST
  Terminator : Terminator
  World1 : sm_lib/Frames and Transforms/World Frame
  Cubesat_RelState : Outport
  wires:
  Constant1/1 -> Product/2
  Cubesat_Acceleration/1 -> Bus Creator/3, Product/1
  Sensor/2(Rel_Velocity) -> Cubesat_Acceleration/2, Bus Creator/2  "Rel_Velocity"
  mean_motion/1 -> Cubesat_Acceleration/3
  Demux/1 -> Simulink-PS Converter1/1
  Sensor/1(Rel_Position) -> Cubesat_Acceleration/1, Bus Creator/1  "Rel_Position"
  Demux/3 -> Simulink-PS Converter3/1
  Demux/2 -> Simulink-PS Converter2/1
  Product/1 -> Add/1
  Thrust/1 -> Add/2
  Add/1 -> Demux/1
  Bus Creator/1 -> Cubesat_RelState/1  "Cubesat_RelState"
  Sensor/3(Rel_Acceleration) -> Terminator/1
  connections:
  6-DOF Joint/LConn4 -- Simulink-PS Converter3/RConn1
  Simulink-PS Converter1/RConn1 -- 6-DOF Joint/LConn2
  Sensor/RConn1 -- 6-DOF Joint/RConn1 -- Brick Solid/RConn1
  6-DOF Joint/LConn3 -- Simulink-PS Converter2/RConn1
  Sensor/LConn1 -- Solver Configuration/RConn1 -- MechanismConfiguration/RConn1 -- World1/RConn1 -- 6-DOF Joint/LConn1

== system SatelliteServicing_Mission/Mission/Cubesat_Inspection/Cubesats/CubeSat1/Zero ==
  Bus Creator3 : BusCreator  Inputs=3
  Constant : Constant  Value=[0,0,0]
  Cubesat_RelState : Outport
  wires:
  Constant/1 -> Bus Creator3/3, Bus Creator3/1, Bus Creator3/2
  Bus Creator3/1 -> Cubesat_RelState/1  "Cubesate_RelState"
